simulink model "sf_stickslip"  (R2017b)
settings: Solver=ode15s  StartTime=0.0  StopTime=20  RelTol=1e-3  AbsTol=1e-6
PreLoadFcn:
  | load('sf_stickslipdat')
undefined symbols (not defined in the file): Fsliding, Fstatic, K, M
libraries: simulink x1
CloseFcn:
  | clear Fsliding  Fstatic   K         M         loaded
settings Model: FPTRunName=Active  ExtModeTrigMode=oneshot  ExtModeArmWhenConnect=off  ExtModeAutoUpdateStatusClock=off  Creator=The MathWorks, Inc.  LastModifiedBy=The MathWorks, Inc.
settings DataIOCC: SaveFormat=Array  SaveState=on
settings OptimizationCC: BooleanDataType=off  ExpressionDepthLimit=2147483647  InitFltsAndDblsToZero=on  LifeSpan=inf
settings DebuggingCC: SaveWithParameterizedLinksMsg=none  UnderspecifiedInitializationDetection=Classic  MergeDetectMultiDrivingBlocksExec=none  SignalResolutionControl=TryResolveAllWithWarning  MultiTaskDSMMsg=warning  MultiTaskCondExecSysMsg=none  IntegerOverflowMsg=none  FcnCallInpInsideContextMsg=warning  StateNameClashWarn=warning  StrictBusMsg=None  SFUnexpectedBacktrackingDiag=warning  SFNoUnconditionalDefaultTransitionDiag=warning  SFExecutionAtInitializationDiag=none  SFMachineParentedDataDiag=none  IntegerSaturationMsg=none
settings HardwareCC: ProdBitPerPointer=32  ProdBitPerSizeT=32  ProdBitPerPtrDiffT=32  ProdLargestAtomicFloat=None  ProdIntDivRoundTo=Undefined  ProdEndianess=Unspecified  ProdWordSize=32  ProdHWDeviceType=32-bit Generic  TargetUnknown=on
settings ModelReferenceCC: PropagateSignalLabelsOutOfModel=off
settings SFSimCC: SimCustomHeaderCode=#include <math.h>  SimParseCustomCode=off
settings CodeAppCC: StateflowObjectComments=on
settings GRTTargetCC: TargetFcnLib=ansi_tfl_tmw.mat  TargetLangStandard=C89/C90 (ANSI)  GeneratePreprocessorConditionals=Disable all  CombineOutputUpdateFcns=off  GRTInterface=on
settings ConfigComp: CovMetricSettings=dcmtr  CovHtmlReporting=on  CovSaveCumulativeToWorkspaceVar=on  CovSaveSingleToWorkspaceVar=on  CovExternalEMLEnable=off  CovSFcnEnable=off

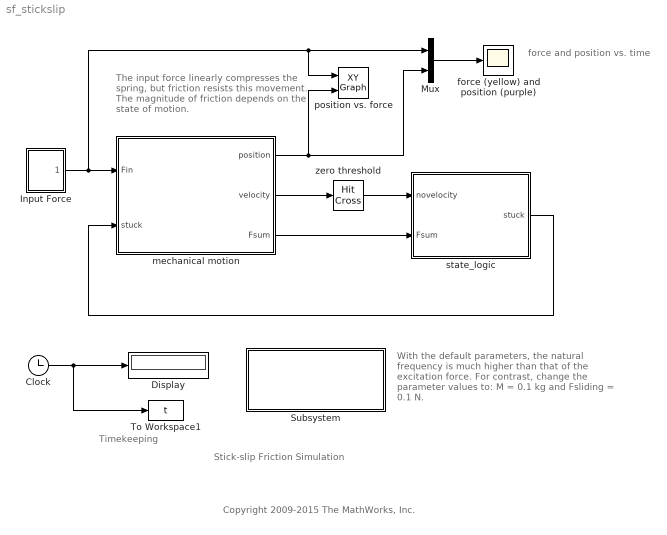
== system sf_stickslip ==
  note: The input force linearly compresses
      | the spring, but friction resists this
      | movement.  The magnitude of
      | friction depends on the state of motion.
  note: force and
      | position
      | vs. time
  note: With the default parameters, the natural
      | frequency is much higher than that of the
      | excitation force.  For contrast, change
      | the parameter values to:
      | M = 0.1 kg and Fsliding = 0.1 N.
  note: Stick-slip Friction Simulation
  note: Timekeeping
  note: Copyright 2009-2015 The MathWorks, Inc.
  Clock : Clock
  Display : Display
  Input Force : Subsystem  mask(Repeating table){rep_seq_t=[0 5 10], rep_seq_y=[0 5 0]}
      mask prompts: rep_seq_t "Time values:"; rep_seq_y "Output values:"
      mask help: Repeating table.
      mask init:
      | period = max(rep_seq_t);
      mask Help: Repeats cycle given in table. Time values should be monotonically increasing.
      mask Display: plot([rep_seq_t,rep_seq_t+period,rep_seq_t+2*period,rep_seq_t(1)+3*period],[rep_seq_y,rep_seq_y,rep_seq_y,rep_seq_y(1)])
  Mux : Mux  Inputs=2
  Subsystem : Subsystem
      settings: OpenFcn=sf_stickslipedit
      mask Display: disp('edit\nparameters')
  To Workspace1 : ToWorkspace  VariableName=t  SampleTime=-1
  force (yellow) and position (purple) : Scope
  mechanical motion : Subsystem
      mask Display: plot(-2,-1,7,3,[0 5],[0 0],[1 1 3 3],[0 2 2 0],[4.5 4.5],[0 3.5],[3 3.25 3.5 3.75 4 4.25 4.5], [1 1 .5  1.5  .5 1 1],[0 1],[1 1],[.5 1 .5],[.5 1 1.5],[0 .5],[-.5 0],[1 1.5],[-.5 0],[2 2.5],[-.5 0],[3 3.5],[-.5 0],[4 5],[-.5 .5],[4.5 5],[1 1.5],[4.5 5],[2 2.5],[4.5 5],[3 3.5],[max(-0.5:0.5:2.5, 1);min(1.5:0.5:4.5,3)],[min(0.5:0.5:3.5, 2); max(-1.5:0.5:1.5, 0)])
  position vs. force : simulink/Sinks/XY Graph  xmin=-1  xmax=6  ymin=-1  ymax=6  st=-1
  state_logic : Stateflow chart  TreatAsAtomicUnit=on
  zero threshold : HitCross
  wires:
  Clock/1 -> Display/1, To Workspace1/1
  Mux/1 -> force (yellow) and position (purple)/1
  zero threshold/1 -> state_logic/1(novelocity)
  mechanical motion/3(Fsum) -> state_logic/2(Fsum)
  mechanical motion/2(velocity) -> zero threshold/1
  mechanical motion/1(position) -> Mux/2, position vs. force/2
  state_logic/1(stuck) -> mechanical motion/2(stuck)
  Input Force/1(out_1) -> mechanical motion/1(Fin), position vs. force/1, Mux/1

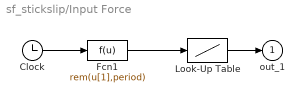
== system sf_stickslip/Input Force ==
  Clock : Clock
  Fcn1 : Fcn  Expr=rem(u[1],period)
  Look-Up Table : Lookup  InputValues=rep_seq_t  Table=rep_seq_y  SaturateOnIntegerOverflow=on
  out_1 : Outport  InitialOutput=0
  wires:
  Look-Up Table/1 -> out_1/1
  Clock/1 -> Fcn1/1
  Fcn1/1 -> Look-Up Table/1

== system sf_stickslip/Subsystem ==

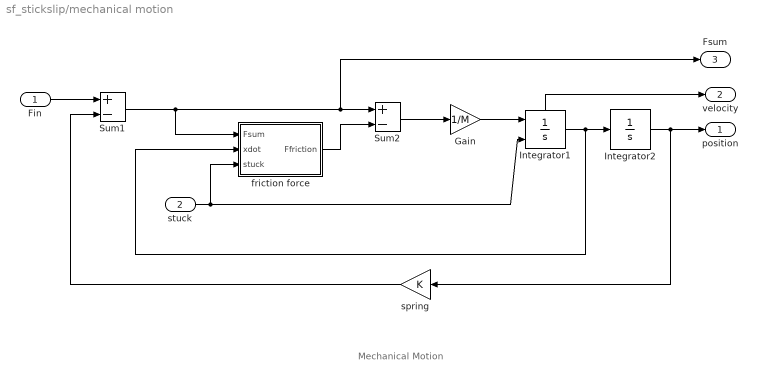
== system sf_stickslip/mechanical motion ==
  note: Mechanical Motion
  Fin : Inport
  stuck : Inport  Port=2
  Gain : Gain  Gain=1/M  SaturateOnIntegerOverflow=on  OutDataTypeStr=Inherit: Same as input  ParamDataTypeStr=Inherit: Same as input
  Integrator1 : Integrator  ExternalReset=rising  ShowStatePort=on
  Integrator2 : Integrator
  Sum1 : Sum  Inputs=+-  SaturateOnIntegerOverflow=on  InputSameDT=on  OutDataTypeStr=Inherit: Same as first input
  Sum2 : Sum  Inputs=+-  SaturateOnIntegerOverflow=on  InputSameDT=on  OutDataTypeStr=Inherit: Same as first input
  friction force : Subsystem
  spring : Gain  Gain=K  SaturateOnIntegerOverflow=on  OutDataTypeStr=Inherit: Same as input  ParamDataTypeStr=Inherit: Same as input
  position : Outport  InitialOutput=0
  velocity : Outport  Port=2  InitialOutput=0
  Fsum : Outport  Port=3  InitialOutput=0
  wires:
  stuck/1 -> friction force/3(stuck), Integrator1/2
  Integrator1/1 -> friction force/2(xdot), Integrator2/1
  Gain/1 -> Integrator1/1
  spring/1 -> Sum1/2
  Sum1/1 -> friction force/1(Fsum), Sum2/1, Fsum/1
  Sum2/1 -> Gain/1
  friction force/1(Ffriction) -> Sum2/2
  Fin/1 -> Sum1/1
  Integrator1/State -> velocity/1
  Integrator2/1 -> spring/1, position/1

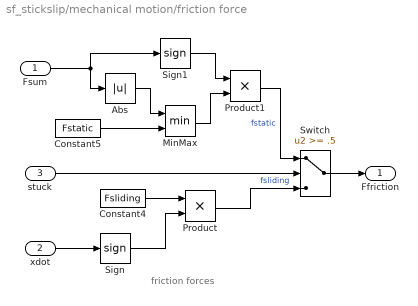
== system sf_stickslip/mechanical motion/friction force ==
  note: friction forces
  Fsum : Inport
  xdot : Inport  Port=2
  stuck : Inport  Port=3
  Abs : Abs  SaturateOnIntegerOverflow=on
  Constant4 : Constant  Value=Fsliding
  Constant5 : Constant  Value=Fstatic
  MinMax : MinMax  Inputs=2  SaturateOnIntegerOverflow=on  InputSameDT=on
  Product : Product  SaturateOnIntegerOverflow=on  RndMeth=Zero  InputSameDT=on  OutDataTypeStr=Inherit: Same as first input
  Product1 : Product  SaturateOnIntegerOverflow=on  RndMeth=Zero  InputSameDT=on  OutDataTypeStr=Inherit: Same as first input
  Sign : Signum
  Sign1 : Signum
  Switch : Switch  Threshold=.5  SaturateOnIntegerOverflow=on  InputSameDT=on
  Ffriction : Outport  InitialOutput=0
  wires:
  Switch/1 -> Ffriction/1
  stuck/1 -> Switch/2
  xdot/1 -> Sign/1
  Sign/1 -> Product/2
  Product/1 -> Switch/3  "fsliding"
  Constant4/1 -> Product/1
  Sign1/1 -> Product1/1
  MinMax/1 -> Product1/2
  Constant5/1 -> MinMax/2
  Abs/1 -> MinMax/1
  Fsum/1 -> Sign1/1, Abs/1
  Product1/1 -> Switch/1  "fstatic"

== stateflow chart sf_stickslip/state_logic ==
  settings: updateMethod=CONTINUOUS
  state state_of_motion
    state sliding/
      entry: stuck = 0;
    state stuck/
      entry: stuck = 1;
    stuck -> sliding : [abs(Fsum) > Fstatic]
    (default) -> stuck
    sliding -> stuck : [novelocity & (abs(Fsum)<= Fstatic)]
  data: stuck output double [0..1]; novelocity input double; Fsum input double
